simulink model "system2"  (R2019a)
settings: Solver=ode1  StartTime=0.0  StopTime=10  FixedStep=0.005  RelTol=1e-3
settings Model: Creator=vmali  LastModifiedBy=vmali

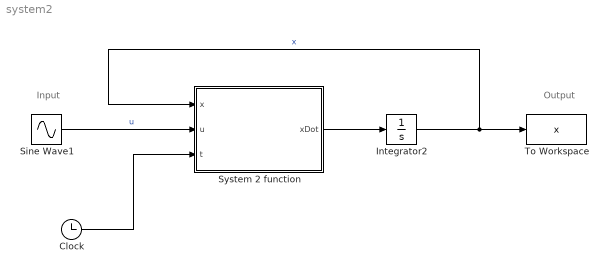
== system system2 ==
  note: Input
  note: Output
  Clock : Clock
      settings: AttributesFormatString=%<Name>
  Integrator2 : Integrator
  Sine Wave1 : Sin  Amplitude=100  Frequency=8*pi  SampleTime=0
      settings: AttributesFormatString=|
      | Amplitude = %<Amplitude>,
      | Frequency = %<Frequency>
  System 2 function : MATLAB Function  TreatAsAtomicUnit=on
  To Workspace : ToWorkspace  VariableName=x  SaveFormat=Structure With Time  SampleTime=-1
      settings: AttributesFormatString=%<Name>
  wires:
  Sine Wave1/1 -> System 2 function/2(u)  "u"
  Integrator2/1 -> To Workspace/1, System 2 function/1(x)  "x"
  System 2 function/1(xDot) -> Integrator2/1
  Clock/1 -> System 2 function/3(t)

== matlab function system2/System 2 function ==
  data: x input; u input; xDot output; t input
function xDot = f(x,u,t)
% Function f of x' = f(x,u,t)
% x == states
% u == inputs

%Give the input parameters

m = 1;
c = 0.5;
k = 30 + 3*sin(2*pi()*t);

% grab memory
xDot = zeros(2,1);

% fill in f of x' = f(x,u,t)
xDot(1) = x(2);
xDot(2) = (1/m)*(u - c*x(2) - k*x(1));
